simulink model "AFE_3L_DCP_DCN"  (R2013b)
settings: Solver=FixedStepDiscrete  SolverMode=SingleTasking  StartTime=0.0  StopTime=0.9  FixedStep=Tpas  RelTol=1e-3
values from neighbouring files (symbols this model uses):
  ASF3 = .5    (= 0.5)    [AFE_FV_Params.m]    (also in AFE_FV_ParamsPV4.m; Params.m)
  Cbus = 330e-3    (= 0.33)    [AFE_FV_Params.m]    (also in AFE_FV_ParamsPV4.m; Params.m)
  DAFE = 0    [AFE_FV_Params.m]    (also in AFE_FV_ParamsPV4.m; Params.m)
  fmod4Q = 1e3    (= 1000)    [AFE_FV_Params.m]    (also in AFE_FV_ParamsPV4.m; Params.m)
  Freq = 50    [AFE_FV_Params.m]    (also in AFE_FV_ParamsPV4.m; Params.m)
  IAFE3L = (PAFE3L+Numd(2)/Dend(1))/Ts    [AFE_FV_Params.m]    (also in AFE_FV_ParamsPV4.m = (PAFE3L+NumdAFE(2)/DendAFE(1))/Ts; CalcPIAndFilters.m; Params.m = (PAFE3L+NumdAFE(2)/DendAFE(1))/Ts)
  IDCP = (PDCP+Numd(2)/Dend(1))/Tpas    [AFE_FV_Params.m]    (also in AFE_FV_ParamsPV4.m = (PDCP+Numd(2)/Dend(1))/Ts; CalcPIAndFilters.m = (PDCP+Numd(2)/Dend(1))/Ts; Params.m = (PDCP+Numd(2)/Dend(1))/Ts)
  Kac = 1/(Vac*sqrt(2/3))    [AFE_FV_Params.m]    (also in AFE_FV_ParamsPV4.m; Params.m)
  KLPDCP = mat2str(KLPDCP)    [CalcPIAndFilters.m]
  L = .1    (= 0.1)    [AFE_FV_Params.m]    (also in AFE_FV_ParamsPV4.m; Params.m)
  Lac = 8.1487e-04    (= 0.00081487)    [AFE_FV_Params.m]    (also in AFE_FV_ParamsPV4.m; Params.m)
  Lcoup = 1e-6    (= 1e-06)    [AFE_FV_Params.m]    (also in AFE_FV_ParamsPV4.m = 1e-05; Params.m = 1e-05)
  NAFE = 100    [AFE_FV_Params.m]    (also in AFE_FV_ParamsPV4.m; Params.m)
  PAFE3L = Numd(1)/Dend(1)    [AFE_FV_Params.m]    (also in AFE_FV_ParamsPV4.m = NumdAFE(1)/DendAFE(1); CalcPIAndFilters.m; Params.m = NumdAFE(1)/DendAFE(1))
  PDCP = Numd(1)/Dend(1)    [AFE_FV_Params.m]    (also in AFE_FV_ParamsPV4.m; CalcPIAndFilters.m; Params.m)
  R = .28    (= 0.28)    [AFE_FV_Params.m]    (also in AFE_FV_ParamsPV4.m; Params.m)
  Sat3 = 800    [AFE_FV_Params.m]
  TLPDCP = mat2str(TLPDCP)    [CalcPIAndFilters.m]
  Tpas = 1e-6    (= 1e-06)    [AFE_FV_Params.m]    (also in AFE_FV_ParamsPV4.m; Params.m = 1e-05)
  Vac = 2000    [AFE_FV_Params.m]    (also in AFE_FV_ParamsPV4.m; Params.m)
  Vdc = 5000    [AFE_FV_Params.m]    (also in AFE_FV_ParamsPV4.m; Params.m)
undefined symbols (not defined in the file or in its folder): D1, Delta, Rac
libraries: powerlib x80, simulink x36, powerlib_meascontrol x26
(part 1 of 2)
settings Model: Creator=LiberT  LastModifiedBy=LiberT
settings DataIOCC: SignalLoggingSaveFormat=ModelDataLogs
settings OptimizationCC: ExpressionDepthLimit=2147483647
settings DebuggingCC: MultiTaskDSMMsg=warning  MultiTaskCondExecSysMsg=none  FcnCallInpInsideContextMsg=EnableAllAsWarning  StateNameClashWarn=warning
settings RTWCC: IncludeERTFirstTime=on

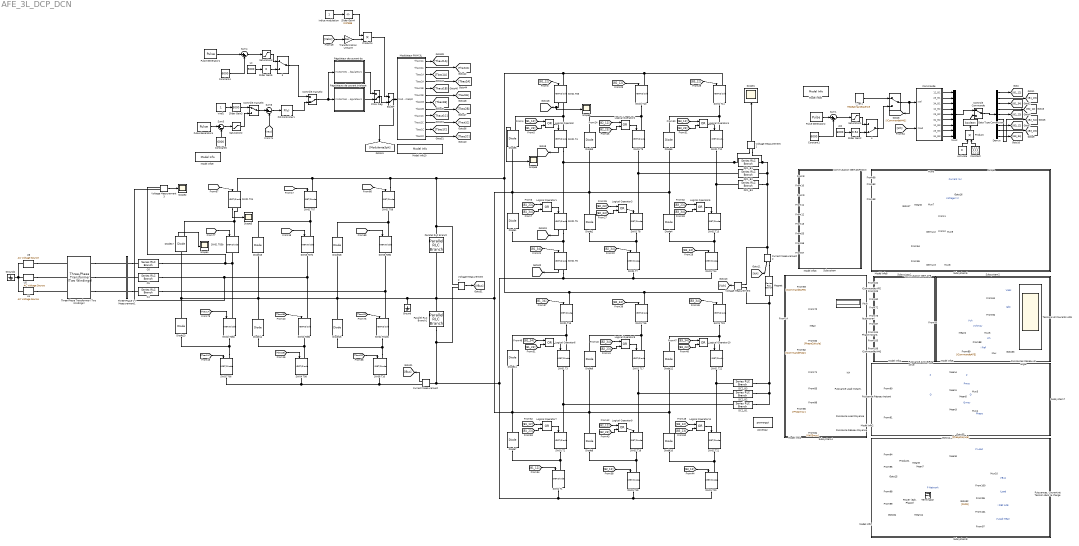
== system AFE_3L_DCP_DCN ==
  " " : ManualSwitch
  " 3" : ManualSwitch
  " 4" : ManualSwitch  CurrentSetting=0
  Activate : Constant  Value=0
  BO/BF : ManualSwitch  CurrentSetting=0
  C4 : powerlib/Elements/Series RLC Branch  LConnTagsString=__new0  RConnTagsString=__new0  BranchType=L  Resistance=Rac  Inductance=Lac  SetiL0=off  InitialCurrent=0  Capacitance=300e-3  Setx0=off  InitialVoltage=0  Measurements=None
  C5 : powerlib/Elements/Series RLC Branch  LConnTagsString=__new0  RConnTagsString=__new0  BranchType=L  Resistance=Rac  Inductance=Lac  SetiL0=off  InitialCurrent=0  Capacitance=300e-3  Setx0=off  InitialVoltage=0  Measurements=None
  C6 : powerlib/Elements/Series RLC Branch  LConnTagsString=__new0  RConnTagsString=__new0  BranchType=L  Resistance=Rac  Inductance=Lac  SetiL0=off  InitialCurrent=0  Capacitance=300e-3  Setx0=off  InitialVoltage=0  Measurements=None
  Choix Reg : ManualSwitch  CurrentSetting=0
  Commande : Subsystem
  Commutation IGBT AFE : Scope  NumInputPorts=9
      settings: TickLabels=on  TimeRange=0.04  YMin=-0.2~-0.2~-0.2~-0.2~-0.2~-0.2~-5~-5~-5  YMax=1.2~1.2~1.2~1.2~1.2~1.2~5~5~5  SaveName=ScopeData4
  Commutation IGBT DCP-DCN : Scope  NumInputPorts=9
      settings: TickLabels=on  TimeRange=0.04  YMin=-0.2~-0.2~-0.2~-0.2~-0.2~-0.2~-0.2~-0.2~-0.2  YMax=1.2~1.2~1.2~1.2~1.2~1.2~1.2~1.2~1.2
  Constant : Constant  Value=[1 1 1 1 1 1 1 1 1]
  Constant1 : Constant  Value=6000
  Constant4 : Constant  Value=6000
  Constant5 : Constant  Value=6000
  Controle Commande : ManualSwitch
  Contrôle manuel2 : ManualSwitch  CurrentSetting=0
  Contrôle manuel3 : ManualSwitch
  Current Measurement : powerlib/Measurements/Current Measurement  PhasorSimulation=off  OutputType=Complex  PSBequivalent=0
  Current Measurement2 : powerlib/Measurements/Current Measurement  PhasorSimulation=off  OutputType=Complex  PSBequivalent=0
  DC1_B1 : powerlib/Elements/Series RLC Branch  LConnTagsString=__new0  RConnTagsString=__new0  BranchType=L  Resistance=0  Inductance=Lcoup  SetiL0=off  InitialCurrent=0  Capacitance=1e-6  Setx0=off  InitialVoltage=0  Measurements=Branch current
  DC1_B2 : powerlib/Elements/Series RLC Branch  LConnTagsString=__new0  RConnTagsString=__new0  BranchType=L  Resistance=0  Inductance=Lcoup  SetiL0=off  InitialCurrent=0  Capacitance=1e-6  Setx0=off  InitialVoltage=0  Measurements=Branch current
  DC1_B3 : powerlib/Elements/Series RLC Branch  LConnTagsString=__new0  RConnTagsString=__new0  BranchType=L  Resistance=0  Inductance=Lcoup  SetiL0=off  InitialCurrent=0  Capacitance=1e-6  Setx0=off  InitialVoltage=0  Measurements=Branch current
  "DC2_B1 " : powerlib/Elements/Series RLC Branch  LConnTagsString=__new0  RConnTagsString=__new0  BranchType=L  Resistance=0  Inductance=Lcoup  SetiL0=off  InitialCurrent=0  Capacitance=1e-6  Setx0=off  InitialVoltage=0  Measurements=Branch current
  DC2_B2 : powerlib/Elements/Series RLC Branch  LConnTagsString=__new0  RConnTagsString=__new0  BranchType=L  Resistance=0  Inductance=Lcoup  SetiL0=off  InitialCurrent=0  Capacitance=1e-6  Setx0=off  InitialVoltage=0  Measurements=Branch current
  DC2_B3 : powerlib/Elements/Series RLC Branch  LConnTagsString=__new0  RConnTagsString=__new0  BranchType=L  Resistance=0  Inductance=Lcoup  SetiL0=off  InitialCurrent=0  Capacitance=1e-6  Setx0=off  InitialVoltage=0  Measurements=Branch current
  Data Type Conversion : DataTypeConversion  OutDataTypeStr=boolean
  Demux : Demux  Outputs=9
  Demux2 : Demux  Outputs=2
  Demux3 : Demux  Outputs=2
  Diode{1..4,6..16,18} (16 alike) : powerlib/Power Electronics/Diode  Ron=0.001  Lon=0  Vf=0.8  IC=0  UseSnubber=off  Rs=500  Cs=inf  Measurements=off
  Diode17 : powerlib/Power Electronics/Diode  Ron=0.001  Lon=0  Vf=0.8  IC=0  UseSnubber=off  Rs=500  Cs=inf  Measurements=on
  Diode5 : powerlib/Power Electronics/Diode  Ron=0.001  Lon=0  Vf=0.8  IC=0  UseSnubber=off  Rs=500  Cs=inf  Measurements=on
  Ground : powerlib/Elements/Ground  LConnTagsString=a
  Ground2 : powerlib/Elements/Ground  LConnTagsString=a
  "ICommande AFE " : Display
  ICommande H4Q : Display
  Ibusmoyen : Display
  Ich : Display
  Logical Operator{,1..11} (12 alike) : Logic  Operator=OR  AllPortsSameDT=off  OutDataTypeStr=boolean
  Magnet : powerlib/Elements/Series RLC Branch  LConnTagsString=__new0  RConnTagsString=__new0  BranchType=RL  Resistance=R  Inductance=L  SetiL0=off  InitialCurrent=0  Capacitance=1e-6  Setx0=off  InitialVoltage=0  Measurements=Branch voltage and current
  Mean{,1..3,8} (5 alike) : powerlib_meascontrol/Measurements/Mean  Freq=50  Vinit=0  Ts=Tpas
  Mean11 : powerlib_meascontrol/Measurements/Mean  Freq=1/.9  Vinit=0  Ts=Tpas
  Mean4 : powerlib_meascontrol/Measurements/Mean  Freq=fmod4Q*3  Vinit=0  Ts=Tpas
  Mean5 : powerlib_meascontrol/Measurements/Mean  Freq=fmod4Q*3  Vinit=0  Ts=Tpas
  Mean6 : powerlib_meascontrol/Measurements/Mean  Freq=fmod4Q/3  Vinit=0  Ts=Tpas
  Mean7 : powerlib_meascontrol/Measurements/Mean  Freq=1/.9  Vinit=0  Ts=Tpas
  Mean9 : powerlib_meascontrol/Measurements/Mean  Freq=fmod4Q/2  Vinit=0  Ts=Tpas
  Model Info{1..5,7..8} (7 alike) : simulink/Model-Wide Utilities/Model Info  InitialBlockCM=None  BlockCM=None  Frame=on  DisplayStringWithTags=Résultats  HorizontalTextAlignment=Center  LeftAlignmentValue=0.5  SourceBlockDiagram=AFE_3L_DCP_DCN  TagMaxNumber=20
  Model Info10 : simulink/Model-Wide Utilities/Model Info  InitialBlockCM=None  BlockCM=None  Frame=on  DisplayStringWithTags=Commande onduleur NPC3L  HorizontalTextAlignment=Center  LeftAlignmentValue=0.5  SourceBlockDiagram=AFE_3L_DCP_DCN  TagMaxNumber=20
  Model Info6 : simulink/Model-Wide Utilities/Model Info  InitialBlockCM=None  BlockCM=None  Frame=on  DisplayStringWithTags=Commande H4Q  HorizontalTextAlignment=Center  LeftAlignmentValue=0.5  SourceBlockDiagram=AFE_3L_DCP_DCN  TagMaxNumber=20
  Model Info9 : simulink/Model-Wide Utilities/Model Info  InitialBlockCM=None  BlockCM=None  Frame=on  DisplayStringWithTags=Commande AFE  HorizontalTextAlignment=Center  LeftAlignmentValue=0.5  SourceBlockDiagram=AFE_3L_DCP_DCN  TagMaxNumber=20
  Modulateur PWM 3L : Subsystem
  Mux{,3..10} (9 alike) : Mux  Inputs=2
  Mux2 : Mux  Inputs=9
  PID Controller1 : simulink/Continuous/PID Controller  Controller=PI  TimeDomain=Discrete-time  SampleTime=Tpas  IntegratorMethod=Forward Euler  FilterMethod=Forward Euler  Form=Parallel  P=PAFE3L  I=IAFE3L  D=0  N=100  InitialConditionSource=internal  InitialConditionForIntegrator=0  InitialConditionForFilter=0  ExternalReset=none  LimitOutput=on  UpperSaturationLimit=Sat3  LowerSaturationLimit=-Sat3  LinearizeAsGain=on  AntiWindupMode=clamping  Kb=1  TrackingMode=off  Kt=1  PParamMin=[]  PParamMax=[]  IParamMin=[]  IParamMax=[]  DParamMin=[]  DParamMax=[]  NParamMin=[]  NParamMax=[]  KbParamMin=[]  KbParamMax=[]  KtParamMin=[]  KtParamMax=[]  POutMin=[]  POutMax=[]  IOutMin=[]  IOutMax=[]  DOutMin=[]  DOutMax=[]  NOutMin=[]  NOutMax=[]  KbOutMin=[]  KbOutMax=[]  KtOutMin=[]  KtOutMax=[]  IntegratorOutMin=[]  IntegratorOutMax=[]  FilterOutMin=[]  FilterOutMax=[]  SumOutMin=[]  SumOutMax=[]  SumI1OutMin=[]  SumI1OutMax=[]  SumI2OutMin=[]  SumI2OutMax=[]  SumI3OutMin=[]  SumI3OutMax=[]  SumDOutMin=[]  SumDOutMax=[]  SaturationOutMin=[]  SaturationOutMax=[]  IntegratorContinuousStateAttributes=''  IntegratorStateMustResolveToSignalObject=off  IntegratorRTWStateStorageClass=Auto  FilterContinuousStateAttributes=''  FilterStateMustResolveToSignalObject=off  FilterRTWStateStorageClass=Auto
  Parallel RLC Branch : powerlib/Elements/Parallel RLC Branch  LConnTagsString=a  RConnTagsString=__new0  BranchType=C  Resistance=9.26  Inductance=1e-3  SetiL0=off  InitialCurrent=0  Capacitance=Cbus*2  Setx0=on  InitialVoltage=Vdc/2  Measurements=None
  Parallel RLC Branch1 : powerlib/Elements/Parallel RLC Branch  LConnTagsString=a  RConnTagsString=__new0  BranchType=C  Resistance=9.26  Inductance=1e-3  SetiL0=off  InitialCurrent=0  Capacitance=Cbus*2  Setx0=on  InitialVoltage=Vdc/2  Measurements=None
  Phase instant. : Display
  "Power (3ph, Phasor)" : powerlib_meascontrol/Measurements/Power (3ph, Phasor)
  Product : Product
  Product1 : Product
  Product4 : Product
  Puissance Active/Reactive : Subsystem
  Puissance Load Instant. : Display
  Puissance Load Moyenne : Display
  Puissance Réseau Instant : Display
  Puissance Réseau Moyenne : Display
  Puissances Réseau et angle : Scope  NumInputPorts=3
      settings: TickLabels=on  TimeRange=0.04  YMin=750000~-400000~-6  YMax=4e+06~250000~10  SaveName=ScopeData2
  "Puissances, Courant et Tension dans la charge" : Scope  NumInputPorts=5
      settings: TickLabels=on  ShowLegends=on  TimeRange=0.9  YMin=2e+06~4650~2000~755~1750  YMax=1.1e+07~5000~4000~800~3250  SaveName=ScopeData7
  Pulse Generator1 : DiscretePulseGenerator  Amplitude=12000  Period=floor(.4/Tpas)  PulseWidth=floor(.4/2/Tpas)  SampleTime=Tpas
  Pulse Generator2 : DiscretePulseGenerator  Amplitude=12000  Period=floor(.4 /Tpas)  PulseWidth=floor(.4 * .5 / Tpas)  PhaseDelay=floor(.001 / Tpas)  SampleTime=Tpas
  Pulse Generator4 : DiscretePulseGenerator  Amplitude=12000  Period=floor(.2/Tpas)  PulseWidth=floor(.2/2/Tpas)  SampleTime=Tpas
  Régulateur de courant dq : Subsystem
  Régulateurs de courant triphasé : Subsystem
  SW01 T05 : powerlib/Power Electronics/IGBT//Diode  Ron=Ron  Rs=Rs  Cs=Cs  Measurements=on
  SW01 T05b : powerlib/Power Electronics/IGBT//Diode  Ron=1e-3  Rs=1e5  Cs=Tpas  Measurements=off
  SW01 T07 : powerlib/Power Electronics/IGBT//Diode  Ron=1e-3  Rs=1e5  Cs=Tpas  Measurements=off
  SW01 T09 : powerlib/Power Electronics/IGBT//Diode  Ron=1e-3  Rs=1e5  Cs=Tpas  Measurements=off
  SW01 T{1..3,7..23} (20 alike) : powerlib/Power Electronics/IGBT//Diode  Ron=Ron  Rs=Rs  Cs=Cs  Measurements=off
  SW01 T24 : powerlib/Power Electronics/IGBT//Diode  Ron=1e-3  Rs=1e5  Cs=Tpas  Measurements=on
  SW01 T4 : powerlib/Power Electronics/IGBT//Diode  Ron=Ron  Rs=Rs  Cs=Cs  Measurements=on
  SW01 T5 : powerlib/Power Electronics/IGBT//Diode  Ron=Ron  Rs=Rs  Cs=Cs  Measurements=on
  SW01 T6 : powerlib/Power Electronics/IGBT//Diode  Ron=Ron  Rs=Rs  Cs=Cs  Measurements=on
  SW02 T010b : powerlib/Power Electronics/IGBT//Diode  Ron=1e-3  Rs=1e5  Cs=Tpas  Measurements=off
  SW02 T06 : powerlib/Power Electronics/IGBT//Diode  Ron=1e-3  Rs=1e5  Cs=Tpas  Measurements=off
  SW02 T06b : powerlib/Power Electronics/IGBT//Diode  Ron=1e-3  Rs=1e5  Cs=Tpas  Measurements=off
  SW02 T08b : powerlib/Power Electronics/IGBT//Diode  Ron=1e-3  Rs=1e5  Cs=Tpas  Measurements=off
  SW03 T07b : powerlib/Power Electronics/IGBT//Diode  Ron=1e-3  Rs=1e5  Cs=Tpas  Measurements=off
  SW04 T08 : powerlib/Power Electronics/IGBT//Diode  Ron=1e-3  Rs=1e5  Cs=Tpas  Measurements=off
  SW05 T09b : powerlib/Power Electronics/IGBT//Diode  Ron=1e-3  Rs=1e5  Cs=Tpas  Measurements=off
  SW06 T10 : powerlib/Power Electronics/IGBT//Diode  Ron=1e-3  Rs=1e5  Cs=Tpas  Measurements=off
  Saturation1 : Saturate  UpperLimit=5000  LowerLimit=2000
  Saturation2 : Saturate  UpperLimit=5500  LowerLimit=4800
  Saturation3 : Saturate  UpperLimit=5000  LowerLimit=1000
  Scope : Scope  NumInputPorts=6
      settings: TimeRange=0.9  YMin=-7000~-5000~-0.1~-0.1~-15000~0  YMax=7000~5000~1.1~1.1~15000~2500  SaveName=hash  MaxDataPoints=10000
  Scope{1..6} (6 alike) : Scope
      Scope1 settings: TimeRange=0.9  YMin=-7000  YMax=7000  SaveName=ScopeData6  MaxDataPoints=10000
      Scope2 settings: YMin=-5500  YMax=5500  SaveName=PHPH
      Scope3 settings: YMin=-1250  YMax=2750  SaveName=IGBTA
      Scope4 settings: YMin=-5500  YMax=5500  SaveName=DIODEA
      Scope5 settings: YMin=-5500  YMax=5500  SaveName=IGBTH
      Scope6 settings: YMin=-5500  YMax=5500  SaveName=DIODEH
  Slider Gain2 : simulink/Math Operations/Slider Gain  low=0  gain=0.54  high=1
  Slider Gain3 : simulink/Math Operations/Slider Gain  low=0  gain=5000  high=7000
  Slider Gain4 : simulink/Math Operations/Slider Gain  low=0  gain=0.97696  high=1
  Slider Gain5 : simulink/Math Operations/Slider Gain  low=0  gain=0  high=1
  Subsystem : Subsystem
      mask Display: disp('')
  Subsystem1 : Subsystem
      mask Display: disp('')
  Subsystem2 : Subsystem
      mask Display: disp('')
  Subsystem4 : Subsystem
      mask Display: disp('')
  Subsystem6 : Subsystem
      mask Display: disp('')
  Subsystem7 : Subsystem
      mask Display: disp('')
  Subsystem8 : Subsystem
      mask Display: disp('')
  Sum{1,4..6} (4 alike) : Sum  Inputs=|+-
  Tensions et Courants AFE : Scope  NumInputPorts=4
      settings: TickLabels=on  ShowLegends=on  TimeRange=0.04  YMin=-2000~-750~4999.4~-800  YMax=2000~750~5000.1~600  SaveName=hach4quadrants
  Terminator : Terminator
  Three-Phase Transformer (Two Windings) : powerlib/Elements/Three-Phase Transformer (Two Windings)  Winding1Connection=Delta (D1)  UNITS=pu  NominalPower=[ 2500e3 , 50 ]  Winding1=[ 18000 , 0 , 0 ]  Winding2Connection=Yg  Winding2=[ 2000 , 0 , 0 ]  SetSaturation=off  Rm=500  Lm=500  Saturation=[ 0,0 ; 0.0024,1.2 ; 1.0,1.52 ]  Hysteresis=off  DataFile='hysteresis'  SetInitialFlux=off  InitialFluxes=[ 0.8 , -0.8 , 0.7 ]  Measurements=None  MoreParameters=off  BreakLoop=off  DataType=off  TransfoNumber=1
  Three-Phase V-I Measurement1 : powerlib/Measurements/Three-Phase V-I Measurement  VoltageMeasurement=phase-to-ground  SetLabelV=on  LabelV=Vabc  Vpu=off  VpuLL=off  CurrentMeasurement=yes  SetLabelI=on  LabelI=Iabc  Ipu=off  Pbase=100e6  Vbase=500e3  OutputType=Complex  PhasorSimulation=off  PSBequivalent=0
  Transformation Unitaire : Gain  Gain=Kac
  U4 : powerlib/Electrical Sources/AC Voltage Source  Amplitude=Vac*sqrt(2/3)*9  Phase=120  Frequency=Freq  SampleTime=Tpas  Measurements=Voltage
  U5 : powerlib/Electrical Sources/AC Voltage Source  Amplitude=Vac*sqrt(2/3)*9  Phase=-120  Frequency=Freq  SampleTime=Tpas  Measurements=Voltage
  U6 : powerlib/Electrical Sources/AC Voltage Source  Amplitude=Vac*sqrt(2/3)*9  Phase=0  Frequency=Freq  SampleTime=Tpas  Measurements=Voltage
  Vbus : Display
  Voltage Measurement{,1..3} (4 alike) : powerlib/Measurements/Voltage Measurement  PhasorSimulation=off  OutputType=Complex  PSBequivalent=0
  Vref1 : Constant  SampleTime=Tpas
  i_ref 1 : simulink/Sources/Repeating Sequence  rep_seq_t="[0 108.51e-3 127.6e-3 132e-3 200e-3 250e-3 283.33e-3 310e-3 366.66e-3  490e-3 533e-3 683.33e-3 900e-3]"  rep_seq_y=[333 333 1000 1031 1500 2000 2500 3000 4000 6000 6000 333 333]
  indice modulation : Constant
  powergui : powerlib/powergui  Priority=1  SimulationMode=Discrete  SolverType=Tustin  SampleTime=Tpas  frequency=60  SPID=off  DisableSnubberDevices=off  DisableRonSwitches=off  DisableVfSwitches=off  SwTol=0  Interpol=off  DisplayEquations=off  frequencyindice=50  Pbase=100e6  ErrMax=1e-4  Iterations=50  UnitsV=kV  UnitsW=MW  FunctionMessages=off  echomessages=off  HookPort=off  EnableUseOfTLC=off  x0status=blocks  RestoreLinks=warning  ResistiveCurrentMeasurement=off  Frange=[0:2:500]  Ylog=off  Xlog=on  ShowGrid=off  save=off  variable=ZData  structure=ScopeData1  ZoomFFT=off  StartTime=18  cycles=100  DisplayStyle=1  fundamental=50  FreqAxis=off  MaxFrequency=2000  frequencyindicesteady=1  RmsSteady=1  display=off  Ts=0  methode=off
  uo : Constant  Value=5000
  uo2 : Constant  Value=6000
  wires:
  [B1_12] -> Commutation IGBT DCP-DCN/1
  [B1_23] -> Commutation IGBT DCP-DCN/2
  [B1_34] -> Commutation IGBT DCP-DCN/3
  [B2_12] -> Commutation IGBT DCP-DCN/4
  [B2_23] -> Commutation IGBT DCP-DCN/5
  [B2_34] -> Commutation IGBT DCP-DCN/6
  Constant/1 -> Product/2
  Activate/1 -> Product/1
  Controle Commande/1 -> Demux/1
  Mux2/1 -> Controle Commande/1
  Data Type Conversion/1 -> Controle Commande/2
  Product/1 -> Data Type Conversion/1
  Demux/1 -> [B1_12]
  Demux/3 -> [B1_34]
  Demux/2 -> [B1_23]
  [B1_12] -> SW01 T05/1
  Logical Operator/1 -> SW01 T4/1
  [B1_12] -> Logical Operator/1
  [B1_23] -> Logical Operator/2
  Logical Operator1/1 -> SW01 T5/1
  [B1_23] -> Logical Operator1/1
  [B1_34] -> Logical Operator1/2
  [B1_34] -> SW01 T6/1
  [B2_12] -> SW01 T10/1
  Logical Operator2/1 -> SW01 T9/1
  [B2_12] -> Logical Operator2/1
  [B2_23] -> Logical Operator2/2
  Logical Operator3/1 -> SW01 T8/1
  [B2_23] -> Logical Operator3/1
  [B2_34] -> Logical Operator3/2
  [B2_34] -> SW01 T7/1
  [B3_12] -> SW01 T11/1
  Logical Operator4/1 -> SW01 T12/1
  [B3_12] -> Logical Operator4/1
  [B3_23] -> Logical Operator4/2
  Logical Operator5/1 -> SW01 T13/1
  [B3_23] -> Logical Operator5/1
  [B3_34] -> Logical Operator5/2
  [B3_34] -> SW01 T14/1
  [B1_34] -> SW01 T15/1
  Logical Operator6/1 -> SW01 T3/1
  [B1_34] -> Logical Operator6/1
  [B1_23] -> Logical Operator6/2
  Logical Operator7/1 -> SW01 T2/1
  [B1_12] -> Logical Operator7/1
  [B1_23] -> Logical Operator7/2
  [B1_12] -> SW01 T1/1
  [B2_34] -> SW01 T16/1
  Logical Operator8/1 -> SW01 T17/1
  [B2_34] -> Logical Operator8/1
  [B2_23] -> Logical Operator8/2
  Logical Operator9/1 -> SW01 T18/1
  [B2_12] -> Logical Operator9/1
  [B2_23] -> Logical Operator9/2
  [B2_12] -> SW01 T19/1
  [B3_34] -> SW01 T23/1
  Logical Operator10/1 -> SW01 T22/1
  [B3_34] -> Logical Operator10/1
  [B3_23] -> Logical Operator10/2
  Logical Operator11/1 -> SW01 T21/1
  [B3_12] -> Logical Operator11/1
  [B3_23] -> Logical Operator11/2
  [B3_12] -> SW01 T20/1
  uo2/1 -> Slider Gain2/1
  Slider Gain2/1 -> " 4"/2
  Saturation1/1 -> " 4"/1
  Constant1/1 -> Sum1/2
  i_ref 1/1 -> " "/1
  " 4"/1 -> " "/2
  Pulse Generator2/1 -> Sum1/1
  Sum1/1 -> Saturation1/1
  " "/1 -> Commande/1(Iref), [ICommandeH4Q]
  Demux/4 -> [B2_12]
  Demux/6 -> [B2_34]
  Demux/5 -> [B2_23]
  Demux/7 -> [B3_12]
  Demux/9 -> [B3_34]
  Demux/8 -> [B3_23]
  Current Measurement2/1 -> [Ich]
  Voltage Measurement/1 -> [Vch]
  [B3_12] -> Commutation IGBT DCP-DCN/7
  [B3_23] -> Commutation IGBT DCP-DCN/8
  [B3_34] -> Commutation IGBT DCP-DCN/9
  Mux6/1 -> [ILoadScope], Scope/1  "Current (A)"
  Mux7/1 -> Scope/2  "Voltage (V)"
  [Ich] -> Mux6/2
  [mIGBT1] -> Demux2/1
  Mean6/1 -> [VMeanLoad], Mux7/2
  [Vch] -> Mux7/1, Mean6/1
  [mIGBT2] -> Demux3/1
  [B1_12] -> Scope/3
  Mux8/1 -> Scope/6
  Mux9/1 -> Scope/5
  [B1_34] -> Scope/4
  Demux2/1 -> Mux9/1
  Demux3/1 -> Mux9/2
  Demux2/2 -> Mux8/1
  Demux3/2 -> Mux8/2
  [ICommandeH4Q] -> Mux6/1
  SW01 T4/1 -> [mIGBT2]
  SW01 T05/1 -> Scope5/1, [mIGBT1]
  SW01 T5/1 -> [mIGBT3]
  SW01 T6/1 -> [mIGBT4]
  Voltage Measurement1/1 -> Scope1/1
  Current Measurement/1 -> [IBus]
  [Thaut1A] -> SW01 T24/1
  [Tbas1A] -> SW02 T06b/1
  [Tbas2A] -> SW02 T06/1
  [Thaut1B] -> SW01 T07/1
  [Thaut2B] -> SW03 T07b/1
  [Tbas1B] -> SW02 T08b/1
  [Tbas2B] -> SW04 T08/1
  [Thaut1C] -> SW01 T09/1
  [Thaut2C] -> SW05 T09b/1
  [Tbas1C] -> SW02 T010b/1
  [Tbas2C] -> SW06 T10/1
  Voltage Measurement2/1 -> [VBus]
  Mean/1 -> Ibusmoyen/1
  [VBus] -> Vbus/1
  [IBus] -> Mean/1
  [ICommandeAFE] -> "ICommande AFE "/1
  [PhaseCalcule] -> Phase instant./1
  [PAFEmoy] -> Puissance Réseau Moyenne/1
  [PH4Q] -> Puissance Load Instant./1
  [Ich] -> Ich/1
  [ICommandeH4Q] -> ICommande H4Q/1
  [PAFE] -> Puissance Réseau Instant/1
  [PH4Qmoy] -> Puissance Load Moyenne/1
  [T5] -> Commutation IGBT AFE/1
  [T56] -> Commutation IGBT AFE/2
  [T6] -> Commutation IGBT AFE/3
  [T7] -> Commutation IGBT AFE/4
  [T78] -> Commutation IGBT AFE/5
  [T8] -> Commutation IGBT AFE/6
  [Vabc] -> Tensions et Courants AFE/1  "Vabc"
  [Iabc] -> Tensions et Courants AFE/2  "Iabc"
  [IBus] -> Mux/1  "Ich"
  [ICommandeAFE] -> Mux/2  "I Ref"
  Mux/1 -> [IBusScope], Tensions et Courants AFE/4
  [Vabc] -> Puissance Active/Reactive/1(Vabc)
  [Iabc] -> Puissance Active/Reactive/2(Iabc)
  Puissance Active/Reactive/1(P) -> Mean4/1, Mean1/1  "P"
  Puissance Active/Reactive/2(Q) -> Mean3/1, Mean5/1  "Q"
  Puissance Active/Reactive/3(PhC) -> Puissances Réseau et angle/3, [PhaseCalcule]  "Phase"
  Mean1/1 -> Mux3/2  "Pmoy"
  Mux3/1 -> Puissances Réseau et angle/1
  Mean3/1 -> Mux4/2  "Qmoy"
  Mux4/1 -> Puissances Réseau et angle/2
  Mux5/1 -> Tensions et Courants AFE/3
  [VBus] -> Mux5/1, Mean2/1  "Vch"
  Mean2/1 -> Mux5/2  "Vchmoy"
  Mean4/1 -> Mux3/1  "P"
  Mean5/1 -> Mux4/1  "Q"
  Mean7/1 -> [PH4Qmoy]
  [Vch] -> Product1/1
  [Ich] -> Product1/2
  Product1/1 -> Mean9/1
  Mean9/1 -> Mean7/1, Mean8/1
  Mean8/1 -> [PH4Q], Mux10/1  "P Load"
  [VMeanLoad] -> "Puissances, Courant et Tension dans la charge"/5  "VLoad Mean"
  Mux10/1 -> "Puissances, Courant et Tension dans la charge"/1
  [VBus] -> "Puissances, Courant et Tension dans la charge"/2  "VBus"
  [ILoadScope] -> "Puissances, Courant et Tension dans la charge"/3  "ILoad"
  [ICommandeAFE] -> "Puissances, Courant et Tension dans la charge"/4  "I REF AFE"
  [Vabc] -> "Power (3ph, Phasor)"/1
  [Iabc] -> "Power (3ph, Phasor)"/2
  Mean11/1 -> [PAFEmoy]
  [T9] -> Commutation IGBT AFE/7
  [T910] -> Commutation IGBT AFE/8
  [T100] -> Commutation IGBT AFE/9
  Commande/1(12_B1) -> Mux2/1
  Commande/2(23_B1) -> Mux2/2
  Commande/3(34_B1) -> Mux2/3
  Commande/4(12_B2) -> Mux2/4
  Commande/5(23_B2) -> Mux2/5
  Commande/6(34_B2) -> Mux2/6
  Commande/7(12_B3) -> Mux2/7
  Commande/8(23_B3) -> Mux2/8
  [Ich] -> Commande/2("Iload ")
  Commande/9(34_B3) -> Mux2/9
  Voltage Measurement3/1 -> Scope2/1
  [Thaut2A] -> SW01 T05b/1
  [VBus] -> Sum6/2
  Vref1/1 -> Slider Gain3/1
  Sum6/1 -> PID Controller1/1
  PID Controller1/1 -> Contrôle manuel2/2
  Contrôle manuel2/1 -> Régulateur de courant dq/1(In1), Régulateurs de courant triphasé/1(In1)
  Sum5/1 -> Saturation2/1
  Pulse Generator4/1 -> Sum5/1
  Constant5/1 -> Sum5/2
  Contrôle manuel3/1 -> Sum6/1
  Slider Gain3/1 -> Contrôle manuel3/1
  Saturation2/1 -> Contrôle manuel3/2
  Modulateur PWM 3L/1(Thaut1A) -> [Thaut1A]
  Modulateur PWM 3L/2(Thaut2A) -> [Thaut2A]
  Modulateur PWM 3L/3(Tbas1A) -> [Tbas1A]
  Modulateur PWM 3L/4(Tbas2A) -> [Tbas2A]
  Modulateur PWM 3L/5(Thaut1B) -> [Thaut1B]
  Modulateur PWM 3L/6(Thaut2B) -> [Thaut2B]
  Modulateur PWM 3L/7(Tbas1B) -> [Tbas1B]
  Modulateur PWM 3L/8(Tbas2B) -> [Tbas2B]
  Modulateur PWM 3L/9(Thaut1C) -> [Thaut1C]
  Modulateur PWM 3L/10(Thaut2C) -> [Thaut2C]
  Modulateur PWM 3L/11(Tbas1C) -> [Tbas1C]
  Modulateur PWM 3L/12(Tbas2C) -> [Tbas2C]
  indice modulation/1 -> Slider Gain4/1
  [Vabc] -> Transformation Unitaire/1
  Transformation Unitaire/1 -> Product4/2
  Slider Gain4/1 -> Product4/1
  BO/BF/1 -> [Modulante3ph], Modulateur PWM 3L/1(Modulante3ph)
  uo/1 -> Slider Gain5/1
  " 3"/1 -> Contrôle manuel2/1
  Slider Gain5/1 -> " 3"/2
  Saturation3/1 -> " 3"/1
  Sum4/1 -> Saturation3/1
  Pulse Generator1/1 -> Sum4/1
  Constant4/1 -> Sum4/2
  Choix Reg/1 -> BO/BF/2
  Régulateurs de courant triphasé/1(Sorties Régulateurs) -> Choix Reg/2
  Régulateur de courant dq/1(Sorties Régulateurs) -> Choix Reg/1
  Product4/1 -> BO/BF/1
  "Power (3ph, Phasor)"/2 -> Terminator/1
  "Power (3ph, Phasor)"/1 -> [PAFE], Mux10/2  "P Network"
  SW01 T24/1 -> Scope3/1
  Diode17/1 -> Scope4/1
  Diode5/1 -> Scope6/1
  connections:
  DC1_B1/LConn1 -- SW01 T5/LConn1 -- SW01 T4/RConn1 -- Voltage Measurement1/LConn1
  DC1_B3/LConn1 -- SW01 T13/LConn1 -- SW01 T12/RConn1
  DC1_B2/LConn1 -- SW01 T9/RConn1 -- SW01 T8/LConn1
  Diode5/RConn1 -- SW01 T05/RConn1 -- SW01 T4/LConn1
  Diode3/RConn1 -- SW01 T10/RConn1 -- SW01 T9/LConn1
  Diode6/RConn1 -- SW01 T12/LConn1 -- SW01 T11/RConn1
  Diode1/LConn1 -- SW01 T6/LConn1 -- SW01 T5/RConn1
  Diode4/LConn1 -- SW01 T14/LConn1 -- SW01 T13/RConn1
  Diode2/LConn1 -- SW01 T8/RConn1 -- SW01 T7/LConn1
  Parallel RLC Branch1/RConn1 -- Voltage Measurement2/LConn2 -- Current Measurement/LConn1 -- SW01 T1/RConn1 -- SW01 T20/RConn1 -- SW01 T19/RConn1 -- SW01 T6/RConn1 -- SW01 T14/RConn1 -- SW01 T7/RConn1
  SW01 T09/LConn1 -- Voltage Measurement2/LConn1 -- Parallel RLC Branch/LConn1 -- SW01 T11/LConn1 -- SW01 T10/LConn1 -- SW01 T05/LConn1 -- SW01 T23/LConn1 -- SW01 T16/LConn1 -- SW01 T15/LConn1 -- SW01 T24/LConn1 -- SW01 T07/LConn1
  Diode11/RConn1 -- SW01 T15/RConn1 -- SW01 T3/LConn1
  Diode9/RConn1 -- SW01 T17/LConn1 -- SW01 T16/RConn1
  Diode12/RConn1 -- SW01 T23/RConn1 -- SW01 T22/LConn1
  Diode7/LConn1 -- SW01 T2/RConn1 -- SW01 T1/LConn1
  Diode10/LConn1 -- SW01 T21/RConn1 -- SW01 T20/LConn1
  Diode8/LConn1 -- SW01 T19/LConn1 -- SW01 T18/RConn1
  Diode13/RConn1 -- Diode17/LConn1 -- Diode15/LConn1 -- Diode14/RConn1 -- Diode16/RConn1 -- Diode18/LConn1 -- Ground/LConn1 -- Parallel RLC Branch1/LConn1 -- Diode11/LConn1 -- Diode7/RConn1 -- Diode9/LConn1 -- Diode8/RConn1 -- Diode10/RConn1 -- Diode12/LConn1 -- Diode4/RConn1 -- Diode6/LConn1 -- Diode3/LConn1 -- Diode2/RConn1 -- Diode5/LConn1 -- Diode1/RConn1 -- Parallel RLC Branch/RConn1
  SW01 T21/LConn1 -- DC2_B3/RConn1 -- SW01 T22/RConn1
  SW01 T2/LConn1 -- "DC2_B1 "/RConn1 -- SW01 T3/RConn1
  SW01 T17/RConn1 -- DC2_B2/RConn1 -- SW01 T18/LConn1
  DC1_B1/RConn1 -- Voltage Measurement/LConn1 -- Current Measurement2/LConn1 -- DC1_B3/RConn1 -- DC1_B2/RConn1 -- Voltage Measurement1/LConn2
  DC2_B3/LConn1 -- "DC2_B1 "/LConn1 -- DC2_B2/LConn1 -- Voltage Measurement/LConn2 -- Magnet/RConn1
  Current Measurement2/RConn1 -- Magnet/LConn1
  C6/LConn1 -- Voltage Measurement3/LConn1 -- SW02 T06b/LConn1 -- SW01 T05b/RConn1
  SW05 T09b/RConn1 -- SW02 T010b/LConn1 -- C4/LConn1
  SW03 T07b/RConn1 -- Voltage Measurement3/LConn2 -- C5/LConn1 -- SW02 T08b/LConn1
  SW01 T24/RConn1 -- SW01 T05b/LConn1 -- Diode17/RConn1
  SW01 T07/RConn1 -- SW03 T07b/LConn1 -- Diode15/RConn1
  SW01 T09/RConn1 -- SW05 T09b/LConn1 -- Diode18/RConn1
  SW02 T06/LConn1 -- SW02 T06b/RConn1 -- Diode13/LConn1
  SW06 T10/LConn1 -- SW02 T010b/RConn1 -- Diode16/LConn1
  SW02 T08b/RConn1 -- SW04 T08/LConn1 -- Diode14/LConn1
  SW04 T08/RConn1 -- SW02 T06/RConn1 -- SW06 T10/RConn1 -- Current Measurement/RConn1
  U5/LConn1 -- Ground2/LConn1 -- U4/LConn1 -- U6/LConn1
  C5/RConn1 -- Three-Phase V-I Measurement1/LConn2
  Three-Phase V-I Measurement1/LConn3 -- C4/RConn1
  U6/RConn1 -- Three-Phase Transformer (Two Windings)/LConn1
  Three-Phase Transformer (Two Windings)/RConn1 -- Three-Phase V-I Measurement1/RConn1
  U5/RConn1 -- Three-Phase Transformer (Two Windings)/LConn2
  Three-Phase Transformer (Two Windings)/RConn2 -- Three-Phase V-I Measurement1/RConn2
  U4/RConn1 -- Three-Phase Transformer (Two Windings)/LConn3
  Three-Phase Transformer (Two Windings)/RConn3 -- Three-Phase V-I Measurement1/RConn3
  Three-Phase V-I Measurement1/LConn1 -- C6/RConn1

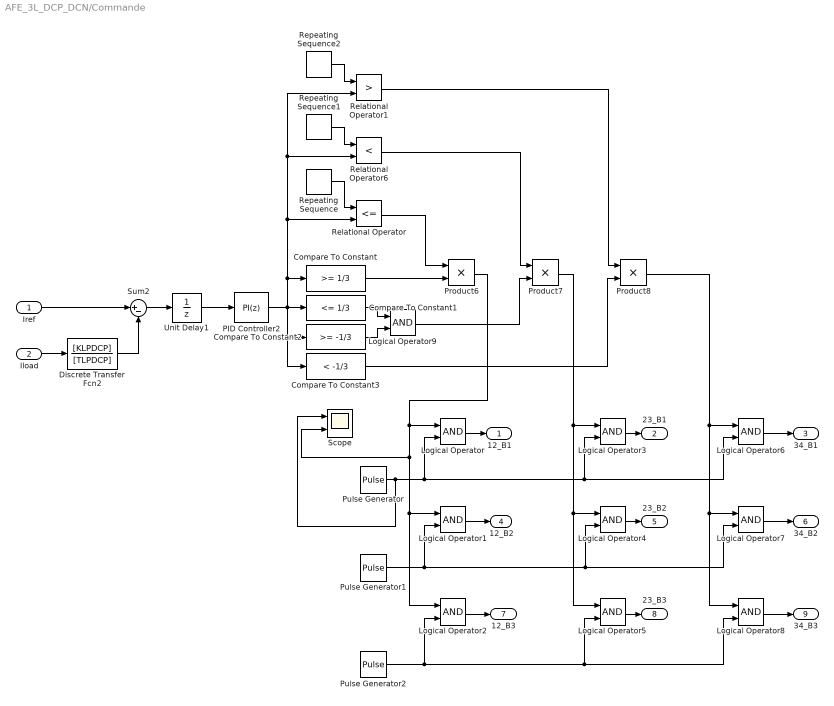
== system AFE_3L_DCP_DCN/Commande ==
  Iref : Inport
  "Iload " : Inport  Port=2
  Compare To Constant : simulink/Logic and Bit Operations/Compare To Constant  relop=>=  const=1/3  OutDataTypeStr=boolean
  Compare To Constant1 : simulink/Logic and Bit Operations/Compare To Constant  relop=<=  const=1/3  OutDataTypeStr=boolean
  Compare To Constant2 : simulink/Logic and Bit Operations/Compare To Constant  relop=>=  const=-1/3  OutDataTypeStr=boolean
  Compare To Constant3 : simulink/Logic and Bit Operations/Compare To Constant  relop=<  const=-1/3  OutDataTypeStr=boolean
  Discrete Transfer Fcn2 : DiscreteTransferFcn  Numerator=[KLPDCP]  Denominator=[TLPDCP]  SampleTime=Tpas
  Logical Operator{,1..9} (10 alike) : Logic  AllPortsSameDT=off  OutDataTypeStr=boolean  SampleTime=Tpas
  PID Controller2 : simulink/Continuous/PID Controller  Controller=PI  TimeDomain=Discrete-time  SampleTime=Tpas  IntegratorMethod=Forward Euler  FilterMethod=Forward Euler  Form=Parallel  P=PDCP  I=IDCP  D=0  N=100  InitialConditionSource=internal  InitialConditionForIntegrator=0  InitialConditionForFilter=0  ExternalReset=none  LimitOutput=on  UpperSaturationLimit=1  LowerSaturationLimit=-1  LinearizeAsGain=on  AntiWindupMode=clamping  Kb=1  TrackingMode=off  Kt=1  PParamMin=[]  PParamMax=[]  IParamMin=[]  IParamMax=[]  DParamMin=[]  DParamMax=[]  NParamMin=[]  NParamMax=[]  KbParamMin=[]  KbParamMax=[]  KtParamMin=[]  KtParamMax=[]  POutMin=[]  POutMax=[]  IOutMin=[]  IOutMax=[]  DOutMin=[]  DOutMax=[]  NOutMin=[]  NOutMax=[]  KbOutMin=[]  KbOutMax=[]  KtOutMin=[]  KtOutMax=[]  IntegratorOutMin=[]  IntegratorOutMax=[]  FilterOutMin=[]  FilterOutMax=[]  SumOutMin=[]  SumOutMax=[]  SumI1OutMin=[]  SumI1OutMax=[]  SumI2OutMin=[]  SumI2OutMax=[]  SumI3OutMin=[]  SumI3OutMax=[]  SumDOutMin=[]  SumDOutMax=[]  SaturationOutMin=[]  SaturationOutMax=[]  IntegratorContinuousStateAttributes=''  IntegratorStateMustResolveToSignalObject=off  IntegratorRTWStateStorageClass=Auto  FilterContinuousStateAttributes=''  FilterStateMustResolveToSignalObject=off  FilterRTWStateStorageClass=Auto
  Product6 : Product  SampleTime=Tpas
  Product7 : Product  SampleTime=Tpas
  Product8 : Product  SampleTime=Tpas
  Pulse Generator : DiscretePulseGenerator  Period=floor(1/(fmod4Q/3) * 1/Tpas)  PulseWidth=floor(1/(fmod4Q) * 1/Tpas)  SampleTime=Tpas
  Pulse Generator1 : DiscretePulseGenerator  Period=floor(1/(fmod4Q/3) * 1/Tpas)  PulseWidth=floor(1/(fmod4Q) * 1/Tpas)  PhaseDelay=floor(1/(fmod4Q) * 1/Tpas)  SampleTime=Tpas
  Pulse Generator2 : DiscretePulseGenerator  Period=floor(1/(fmod4Q/3) * 1/Tpas)  PulseWidth=floor(1/(fmod4Q) * 1/Tpas)  PhaseDelay=floor(2/(fmod4Q) * 1/Tpas)  SampleTime=Tpas
  Relational Operator : RelationalOperator  Operator=<=  OutDataTypeStr=boolean
  Relational Operator1 : RelationalOperator  Operator=>  OutDataTypeStr=boolean
  Relational Operator6 : RelationalOperator  Operator=<  OutDataTypeStr=boolean
  Repeating Sequence : simulink/Sources/Repeating Sequence  rep_seq_t=[0 1/fmod4Q]  rep_seq_y=[1/3 1.035]
  Repeating Sequence1 : simulink/Sources/Repeating Sequence  rep_seq_t=[0 1/fmod4Q]  rep_seq_y=[-.35 .35]
  Repeating Sequence2 : simulink/Sources/Repeating Sequence  rep_seq_t=[0 1/fmod4Q]  rep_seq_y=[-1 -1/3]
  Scope : Scope  NumInputPorts=2
      settings: YMin=-5~-5  YMax=5~5  SaveName=aaaaa
  Sum2 : Sum  Inputs=|+-
  Unit Delay1 : UnitDelay  SampleTime=-1
  12_B1 : Outport
  23_B1 : Outport  Port=2
  34_B1 : Outport  Port=3
  12_B2 : Outport  Port=4
  23_B2 : Outport  Port=5
  34_B2 : Outport  Port=6
  12_B3 : Outport  Port=7
  23_B3 : Outport  Port=8
  34_B3 : Outport  Port=9
  wires:
  Compare To Constant/1 -> Product6/2
  Compare To Constant3/1 -> Product8/2
  Compare To Constant1/1 -> Logical Operator9/1
  Compare To Constant2/1 -> Logical Operator9/2
  Logical Operator9/1 -> Product7/2
  Repeating Sequence/1 -> Relational Operator/1
  Repeating Sequence2/1 -> Relational Operator1/1
  Relational Operator/1 -> Product6/1
  Relational Operator6/1 -> Product7/1
  Relational Operator1/1 -> Product8/1
  PID Controller2/1 -> Relational Operator/2, Relational Operator1/2, Relational Operator6/2, Compare To Constant/1, Compare To Constant1/1, Compare To Constant3/1, Compare To Constant2/1
  Repeating Sequence1/1 -> Relational Operator6/1
  Iref/1 -> Sum2/1
  "Iload "/1 -> Discrete Transfer Fcn2/1
  Discrete Transfer Fcn2/1 -> Sum2/2
  Sum2/1 -> Unit Delay1/1
  Unit Delay1/1 -> PID Controller2/1
  Product6/1 -> Scope/2, Logical Operator2/1, Logical Operator1/1, Logical Operator/1
  Pulse Generator2/1 -> Logical Operator5/2, Logical Operator8/2, Logical Operator2/2
  Pulse Generator/1 -> Scope/1, Logical Operator3/2, Logical Operator6/2, Logical Operator/2
  Pulse Generator1/1 -> Logical Operator1/2, Logical Operator4/2, Logical Operator7/2
  Product7/1 -> Logical Operator5/1, Logical Operator4/1, Logical Operator3/1
  Product8/1 -> Logical Operator8/1, Logical Operator7/1, Logical Operator6/1
  Logical Operator/1 -> 12_B1/1
  Logical Operator8/1 -> 34_B3/1
  Logical Operator1/1 -> 12_B2/1
  Logical Operator3/1 -> 23_B1/1
  Logical Operator6/1 -> 34_B1/1
  Logical Operator2/1 -> 12_B3/1
  Logical Operator5/1 -> 23_B3/1
  Logical Operator7/1 -> 34_B2/1
  Logical Operator4/1 -> 23_B2/1

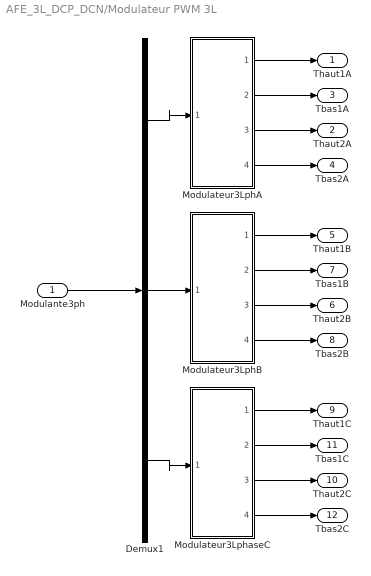
== system AFE_3L_DCP_DCN/Modulateur PWM 3L ==
  Modulante3ph : Inport
  Demux1 : Demux  Outputs=3
  "Modulateur3LphA " : Subsystem
  Modulateur3LphB : Subsystem
  Modulateur3LphaseC : Subsystem
  Thaut1A : Outport
  Thaut2A : Outport  Port=2
  Tbas1A : Outport  Port=3
  Tbas2A : Outport  Port=4
  Thaut1B : Outport  Port=5
  Thaut2B : Outport  Port=6
  Tbas1B : Outport  Port=7
  Tbas2B : Outport  Port=8
  Thaut1C : Outport  Port=9
  Thaut2C : Outport  Port=10
  Tbas1C : Outport  Port=11
  Tbas2C : Outport  Port=12
  wires:
  Modulante3ph/1 -> Demux1/1
  Demux1/1 -> "Modulateur3LphA "/1(Modulante)
  "Modulateur3LphA "/1(Thaut1) -> Thaut1A/1
  "Modulateur3LphA "/2(Tbas1) -> Tbas1A/1
  "Modulateur3LphA "/3(Thaut2) -> Thaut2A/1
  "Modulateur3LphA "/4(Tbas2) -> Tbas2A/1
  Demux1/2 -> Modulateur3LphB/1(Modulante)
  Modulateur3LphB/1(Thaut1) -> Thaut1B/1
  Modulateur3LphB/2(Tbas1) -> Tbas1B/1
  Modulateur3LphB/3(Thaut2) -> Thaut2B/1
  Modulateur3LphB/4(Tbas2) -> Tbas2B/1
  Demux1/3 -> Modulateur3LphaseC/1(Modulante)
  Modulateur3LphaseC/1(Thaut1) -> Thaut1C/1
  Modulateur3LphaseC/2(Tbas1) -> Tbas1C/1
  Modulateur3LphaseC/3(Thaut2) -> Thaut2C/1
  Modulateur3LphaseC/4(Tbas2) -> Tbas2C/1

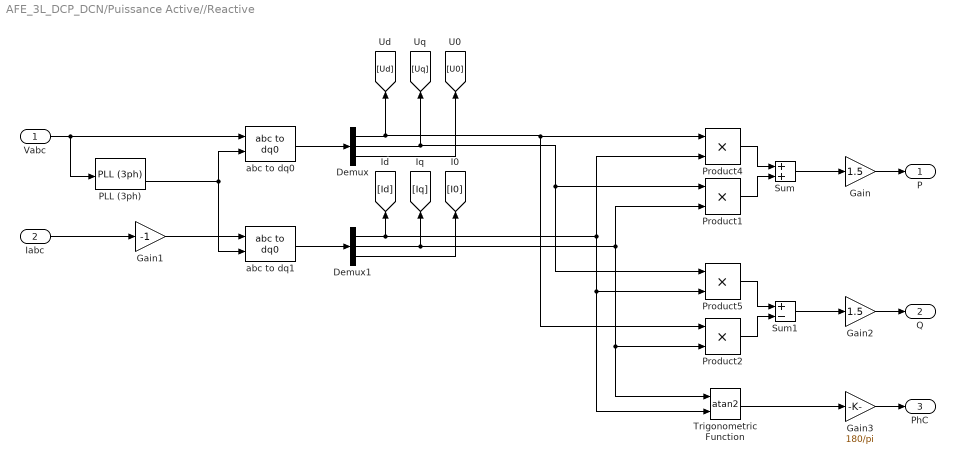
== system AFE_3L_DCP_DCN/Puissance Active//Reactive ==
  Vabc : Inport
  Iabc : Inport  Port=2
  Demux : Demux  Outputs=3
  Demux1 : Demux  Outputs=3
  Gain : Gain  Gain=1.5
  Gain1 : Gain  Gain=-1
  Gain2 : Gain  Gain=1.5
  Gain3 : Gain  Gain=180/pi
  PLL (3ph) : powerlib_meascontrol/PLL/PLL (3ph)  Fmin=49  Par_Init=[0, 50]  ParK=[180, 3200, 1]  TcD=1e-4  MaxRateChangeFreq=6  FilterCutOffFreq=25  Ts=Tpas  AGC=on
  Product{1..2,4..5} (4 alike) : Product
  Sum : Sum
  Sum1 : Sum  Inputs=+-
  Trigonometric Function : Trigonometry  Operator=atan2
  abc to dq0 : powerlib_meascontrol/Transformations/abc to dq0  Alignment=90 degrees behind phase A axis
  abc to dq1 : powerlib_meascontrol/Transformations/abc to dq0  Alignment=90 degrees behind phase A axis
  P : Outport
  Q : Outport  Port=2
  PhC : Outport  Port=3
  wires:
  Vabc/1 -> PLL (3ph)/1, abc to dq0/1
  abc to dq0/1 -> Demux/1
  abc to dq1/1 -> Demux1/1
  Product2/1 -> Sum1/2
  Sum1/1 -> Gain2/1
  Demux/3 -> [U0]
  Demux/2 -> Product5/1, Product1/1, [Uq]
  Demux/1 -> Product2/1, Product4/1, [Ud]
  Demux1/2 -> [Iq], Trigonometric Function/1, Product2/2, Product1/2
  Product5/1 -> Sum1/1
  Gain2/1 -> Q/1
  Trigonometric Function/1 -> Gain3/1
  Gain3/1 -> PhC/1
  Product4/1 -> Sum/1
  Product1/1 -> Sum/2
  Sum/1 -> Gain/1
  Gain/1 -> P/1
  Demux1/1 -> [Id], Trigonometric Function/2, Product5/2, Product4/2
  Demux1/3 -> [I0]
  PLL (3ph)/2 -> abc to dq1/2, abc to dq0/2
  Iabc/1 -> Gain1/1
  Gain1/1 -> abc to dq1/1

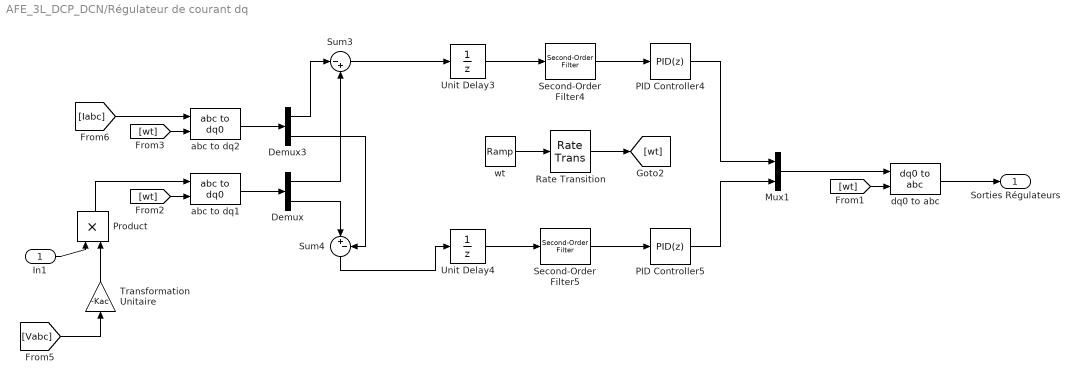
== system AFE_3L_DCP_DCN/Régulateur de courant dq ==
  In1 : Inport
  Demux : Demux  Outputs=2
  Demux3 : Demux  Outputs=2
  Mux1 : Mux  Inputs=2
  PID Controller4 : simulink/Continuous/PID Controller  Controller=PID  TimeDomain=Discrete-time  SampleTime=Tpas  IntegratorMethod=Forward Euler  FilterMethod=Forward Euler  Form=Parallel  P=PAFE3L  I=IAFE3L  D=DAFE  N=NAFE  InitialConditionSource=internal  InitialConditionForIntegrator=0  InitialConditionForFilter=0  ExternalReset=none  LimitOutput=on  UpperSaturationLimit=0.95  LowerSaturationLimit=-0.95  LinearizeAsGain=on  AntiWindupMode=clamping  Kb=1  TrackingMode=off  Kt=1  PParamMin=[]  PParamMax=[]  IParamMin=[]  IParamMax=[]  DParamMin=[]  DParamMax=[]  NParamMin=[]  NParamMax=[]  KbParamMin=[]  KbParamMax=[]  KtParamMin=[]  KtParamMax=[]  POutMin=[]  POutMax=[]  IOutMin=[]  IOutMax=[]  DOutMin=[]  DOutMax=[]  NOutMin=[]  NOutMax=[]  KbOutMin=[]  KbOutMax=[]  KtOutMin=[]  KtOutMax=[]  IntegratorOutMin=[]  IntegratorOutMax=[]  FilterOutMin=[]  FilterOutMax=[]  SumOutMin=[]  SumOutMax=[]  SumI1OutMin=[]  SumI1OutMax=[]  SumI2OutMin=[]  SumI2OutMax=[]  SumI3OutMin=[]  SumI3OutMax=[]  SumDOutMin=[]  SumDOutMax=[]  SaturationOutMin=[]  SaturationOutMax=[]  IntegratorContinuousStateAttributes=''  IntegratorStateMustResolveToSignalObject=off  IntegratorRTWStateStorageClass=Auto  FilterContinuousStateAttributes=''  FilterStateMustResolveToSignalObject=off  FilterRTWStateStorageClass=Auto
  PID Controller5 : simulink/Continuous/PID Controller  Controller=PID  TimeDomain=Discrete-time  SampleTime=Tpas  IntegratorMethod=Forward Euler  FilterMethod=Forward Euler  Form=Parallel  P=PAFE3L  I=IAFE3L  D=DAFE  N=NAFE  InitialConditionSource=internal  InitialConditionForIntegrator=0  InitialConditionForFilter=0  ExternalReset=none  LimitOutput=on  UpperSaturationLimit=0.95  LowerSaturationLimit=-0.95  LinearizeAsGain=on  AntiWindupMode=clamping  Kb=1  TrackingMode=off  Kt=1  PParamMin=[]  PParamMax=[]  IParamMin=[]  IParamMax=[]  DParamMin=[]  DParamMax=[]  NParamMin=[]  NParamMax=[]  KbParamMin=[]  KbParamMax=[]  KtParamMin=[]  KtParamMax=[]  POutMin=[]  POutMax=[]  IOutMin=[]  IOutMax=[]  DOutMin=[]  DOutMax=[]  NOutMin=[]  NOutMax=[]  KbOutMin=[]  KbOutMax=[]  KtOutMin=[]  KtOutMax=[]  IntegratorOutMin=[]  IntegratorOutMax=[]  FilterOutMin=[]  FilterOutMax=[]  SumOutMin=[]  SumOutMax=[]  SumI1OutMin=[]  SumI1OutMax=[]  SumI2OutMin=[]  SumI2OutMax=[]  SumI3OutMin=[]  SumI3OutMax=[]  SumDOutMin=[]  SumDOutMax=[]  SaturationOutMin=[]  SaturationOutMax=[]  IntegratorContinuousStateAttributes=''  IntegratorStateMustResolveToSignalObject=off  IntegratorRTWStateStorageClass=Auto  FilterContinuousStateAttributes=''  FilterStateMustResolveToSignalObject=off  FilterRTWStateStorageClass=Auto
  Product : Product
  Rate Transition : RateTransition  OutPortSampleTime=Ts
  Second-Order Filter4 : powerlib_meascontrol/Filters/Second-Order Filter  FilterType=Lowpass  Fo=ASF3*fmod4Q  Zeta=QSF3  Ts=Tpas  Initialize=on  Vac_Init="[0,  0,  50]"  Vdc_Init=0  PlotResponse=off  FreqRange=[0, 10000, 1]
  Second-Order Filter5 : powerlib_meascontrol/Filters/Second-Order Filter  FilterType=Lowpass  Fo=ASF3*fmod4Q  Zeta=QSF3  Ts=Tpas  Initialize=on  Vac_Init="[0,  0,  50]"  Vdc_Init=0  PlotResponse=off  FreqRange=[0, 10000, 1]
  Sum3 : Sum  Inputs=|-+
  Sum4 : Sum  Inputs=|+-
  Transformation Unitaire : Gain  Gain=-Kac
  Unit Delay3 : UnitDelay  SampleTime=-1
  Unit Delay4 : UnitDelay  SampleTime=-1
  abc to dq1 : powerlib_meascontrol/Transformations/abc to dq0  Alignment=Aligned with phase A axis
  abc to dq2 : powerlib_meascontrol/Transformations/abc to dq0  Alignment=Aligned with phase A axis
  dq0 to abc : powerlib_meascontrol/Transformations/dq0 to abc  Alignment=Aligned with phase A axis
  wt : simulink/Sources/Ramp  slope=2*pi*50  start=0  X0=0
  Sorties Régulateurs : Outport
  wires:
  [Vabc] -> Transformation Unitaire/1
  Transformation Unitaire/1 -> Product/2
  In1/1 -> Product/1
  abc to dq1/1 -> Demux/1
  [wt] -> abc to dq1/2
  [wt] -> dq0 to abc/2
  wt/1 -> Rate Transition/1
  Rate Transition/1 -> [wt]
  Mux1/1 -> dq0 to abc/1
  Sum3/1 -> Unit Delay3/1
  PID Controller4/1 -> Mux1/1
  Demux/1 -> Sum3/2
  [Iabc] -> abc to dq2/1
  [wt] -> abc to dq2/2
  abc to dq2/1 -> Demux3/1
  Demux3/1 -> Sum3/1
  Product/1 -> abc to dq1/1
  Sum4/1 -> Unit Delay4/1
  PID Controller5/1 -> Mux1/2
  dq0 to abc/1 -> Sorties Régulateurs/1
  Unit Delay3/1 -> Second-Order Filter4/1
  Second-Order Filter4/1 -> PID Controller4/1
  Unit Delay4/1 -> Second-Order Filter5/1
  Second-Order Filter5/1 -> PID Controller5/1
  Demux/2 -> Sum4/1
  Demux3/2 -> Sum4/2

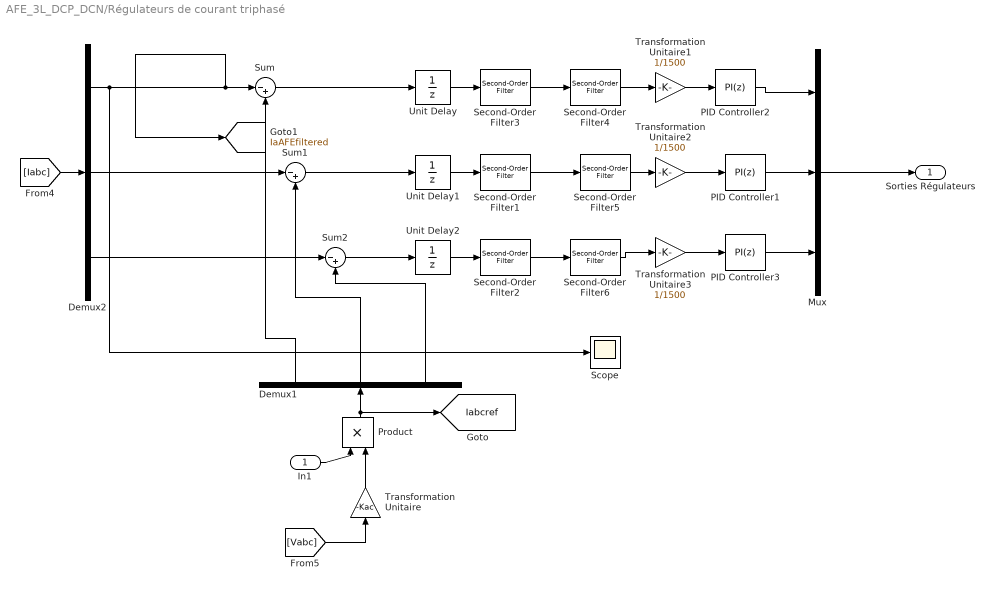
== system AFE_3L_DCP_DCN/Régulateurs de courant triphasé ==
  In1 : Inport
  Demux1 : Demux  Outputs=3
  Demux2 : Demux  Outputs=3
  Mux : Mux  Inputs=3
  PID Controller1 : simulink/Continuous/PID Controller  Controller=PI  TimeDomain=Discrete-time  SampleTime=Tpas  IntegratorMethod=Forward Euler  FilterMethod=Forward Euler  Form=Parallel  P=PDCP  I=IDCP  D=DAFE  N=NAFE  InitialConditionSource=internal  InitialConditionForIntegrator=0  InitialConditionForFilter=0  ExternalReset=none  LimitOutput=on  UpperSaturationLimit=0.95  LowerSaturationLimit=-0.95  LinearizeAsGain=on  AntiWindupMode=clamping  Kb=1  TrackingMode=off  Kt=1  PParamMin=[]  PParamMax=[]  IParamMin=[]  IParamMax=[]  DParamMin=[]  DParamMax=[]  NParamMin=[]  NParamMax=[]  KbParamMin=[]  KbParamMax=[]  KtParamMin=[]  KtParamMax=[]  POutMin=[]  POutMax=[]  IOutMin=[]  IOutMax=[]  DOutMin=[]  DOutMax=[]  NOutMin=[]  NOutMax=[]  KbOutMin=[]  KbOutMax=[]  KtOutMin=[]  KtOutMax=[]  IntegratorOutMin=[]  IntegratorOutMax=[]  FilterOutMin=[]  FilterOutMax=[]  SumOutMin=[]  SumOutMax=[]  SumI1OutMin=[]  SumI1OutMax=[]  SumI2OutMin=[]  SumI2OutMax=[]  SumI3OutMin=[]  SumI3OutMax=[]  SumDOutMin=[]  SumDOutMax=[]  SaturationOutMin=[]  SaturationOutMax=[]  IntegratorContinuousStateAttributes=''  IntegratorStateMustResolveToSignalObject=off  IntegratorRTWStateStorageClass=Auto  FilterContinuousStateAttributes=''  FilterStateMustResolveToSignalObject=off  FilterRTWStateStorageClass=Auto
  PID Controller2 : simulink/Continuous/PID Controller  Controller=PI  TimeDomain=Discrete-time  SampleTime=Tpas  IntegratorMethod=Forward Euler  FilterMethod=Forward Euler  Form=Parallel  P=PDCP  I=IDCP  D=DAFE  N=NAFE  InitialConditionSource=internal  InitialConditionForIntegrator=0  InitialConditionForFilter=0  ExternalReset=none  LimitOutput=on  UpperSaturationLimit=0.95  LowerSaturationLimit=-0.95  LinearizeAsGain=on  AntiWindupMode=clamping  Kb=1  TrackingMode=off  Kt=1  PParamMin=[]  PParamMax=[]  IParamMin=[]  IParamMax=[]  DParamMin=[]  DParamMax=[]  NParamMin=[]  NParamMax=[]  KbParamMin=[]  KbParamMax=[]  KtParamMin=[]  KtParamMax=[]  POutMin=[]  POutMax=[]  IOutMin=[]  IOutMax=[]  DOutMin=[]  DOutMax=[]  NOutMin=[]  NOutMax=[]  KbOutMin=[]  KbOutMax=[]  KtOutMin=[]  KtOutMax=[]  IntegratorOutMin=[]  IntegratorOutMax=[]  FilterOutMin=[]  FilterOutMax=[]  SumOutMin=[]  SumOutMax=[]  SumI1OutMin=[]  SumI1OutMax=[]  SumI2OutMin=[]  SumI2OutMax=[]  SumI3OutMin=[]  SumI3OutMax=[]  SumDOutMin=[]  SumDOutMax=[]  SaturationOutMin=[]  SaturationOutMax=[]  IntegratorContinuousStateAttributes=''  IntegratorStateMustResolveToSignalObject=off  IntegratorRTWStateStorageClass=Auto  FilterContinuousStateAttributes=''  FilterStateMustResolveToSignalObject=off  FilterRTWStateStorageClass=Auto
  PID Controller3 : simulink/Continuous/PID Controller  Controller=PI  TimeDomain=Discrete-time  SampleTime=Tpas  IntegratorMethod=Forward Euler  FilterMethod=Forward Euler  Form=Parallel  P=PDCP  I=IDCP  D=DAFE  N=NAFE  InitialConditionSource=internal  InitialConditionForIntegrator=0  InitialConditionForFilter=0  ExternalReset=none  LimitOutput=on  UpperSaturationLimit=0.95  LowerSaturationLimit=-0.95  LinearizeAsGain=on  AntiWindupMode=clamping  Kb=1  TrackingMode=off  Kt=1  PParamMin=[]  PParamMax=[]  IParamMin=[]  IParamMax=[]  DParamMin=[]  DParamMax=[]  NParamMin=[]  NParamMax=[]  KbParamMin=[]  KbParamMax=[]  KtParamMin=[]  KtParamMax=[]  POutMin=[]  POutMax=[]  IOutMin=[]  IOutMax=[]  DOutMin=[]  DOutMax=[]  NOutMin=[]  NOutMax=[]  KbOutMin=[]  KbOutMax=[]  KtOutMin=[]  KtOutMax=[]  IntegratorOutMin=[]  IntegratorOutMax=[]  FilterOutMin=[]  FilterOutMax=[]  SumOutMin=[]  SumOutMax=[]  SumI1OutMin=[]  SumI1OutMax=[]  SumI2OutMin=[]  SumI2OutMax=[]  SumI3OutMin=[]  SumI3OutMax=[]  SumDOutMin=[]  SumDOutMax=[]  SaturationOutMin=[]  SaturationOutMax=[]  IntegratorContinuousStateAttributes=''  IntegratorStateMustResolveToSignalObject=off  IntegratorRTWStateStorageClass=Auto  FilterContinuousStateAttributes=''  FilterStateMustResolveToSignalObject=off  FilterRTWStateStorageClass=Auto
  Product : Product
  Scope : Scope
      settings: TimeRange=0.04  YMin=-6000  YMax=6000  SaveName=ScopeData2
  Second-Order Filter{1..6} (6 alike) : powerlib_meascontrol/Filters/Second-Order Filter  FilterType=Lowpass  Fo=1.25*fmod4Q  Zeta=1  Ts=Tpas  Initialize=on  Vac_Init="[0,  0,  50]"  Vdc_Init=0  PlotResponse=off  FreqRange=[0, 10000, 1]
  Sum : Sum  Inputs=|-+
  Sum1 : Sum  Inputs=|-+
  Sum2 : Sum  Inputs=|-+
  Transformation Unitaire : Gain  Gain=-Kac
  Transformation Unitaire1 : Gain  Gain=1/1500
  Transformation Unitaire2 : Gain  Gain=1/1500
  Transformation Unitaire3 : Gain  Gain=1/1500
  Unit Delay : UnitDelay  SampleTime=-1
  Unit Delay1 : UnitDelay  SampleTime=-1
  Unit Delay2 : UnitDelay  SampleTime=-1
  Sorties Régulateurs : Outport
  tag scope: IaAFEfiltered=global, Iabcref=global
  wires:
  Sum/1 -> Unit Delay/1
  Sum1/1 -> Unit Delay1/1
  Sum2/1 -> Unit Delay2/1
  [Iabc] -> Demux2/1
  [Vabc] -> Transformation Unitaire/1
  Demux1/1 -> Sum/2
  Demux1/2 -> Sum1/2
  Demux1/3 -> Sum2/2
  Transformation Unitaire/1 -> Product/2
  In1/1 -> Product/1
  Product/1 -> Demux1/1, [Iabcref]
  PID Controller3/1 -> Mux/3
  PID Controller1/1 -> Mux/2
  PID Controller2/1 -> Mux/1
  Demux2/1 -> [IaAFEfiltered], Sum/1, Scope/1
  Demux2/2 -> Sum1/1
  Demux2/3 -> Sum2/1
  Second-Order Filter3/1 -> Second-Order Filter4/1
  Unit Delay/1 -> Second-Order Filter3/1
  Unit Delay1/1 -> Second-Order Filter1/1
  Second-Order Filter1/1 -> Second-Order Filter5/1
  Second-Order Filter2/1 -> Second-Order Filter6/1
  Unit Delay2/1 -> Second-Order Filter2/1
  Mux/1 -> Sorties Régulateurs/1
  Second-Order Filter4/1 -> Transformation Unitaire1/1
  Second-Order Filter5/1 -> Transformation Unitaire2/1
  Second-Order Filter6/1 -> Transformation Unitaire3/1
  Transformation Unitaire1/1 -> PID Controller2/1
  Transformation Unitaire2/1 -> PID Controller1/1
  Transformation Unitaire3/1 -> PID Controller3/1

== system AFE_3L_DCP_DCN/Subsystem ==

== system AFE_3L_DCP_DCN/Subsystem1 ==

== system AFE_3L_DCP_DCN/Subsystem2 ==

== system AFE_3L_DCP_DCN/Subsystem4 ==

== system AFE_3L_DCP_DCN/Subsystem6 ==

== system AFE_3L_DCP_DCN/Subsystem7 ==

== system AFE_3L_DCP_DCN/Subsystem8 ==

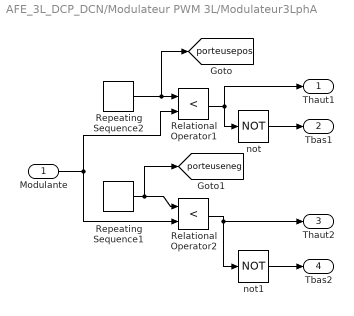
== system AFE_3L_DCP_DCN/Modulateur PWM 3L/Modulateur3LphA  ==
  Modulante : Inport
  Relational Operator1 : RelationalOperator  Operator=<  OutDataTypeStr=boolean
  Relational Operator2 : RelationalOperator  Operator=<  OutDataTypeStr=boolean
  Repeating Sequence1 : simulink/Sources/Repeating Sequence  rep_seq_t=[0 .5/(666) 1/(666)]  rep_seq_y=[-1 0 -1]
  Repeating Sequence2 : simulink/Sources/Repeating Sequence  rep_seq_t=[0 .5/(666) 1/(666)]  rep_seq_y=[0 1 0]
  not : Logic  Operator=NOT  IconShape=distinctive  AllPortsSameDT=off  OutDataTypeStr=boolean
  not1 : Logic  Operator=NOT  IconShape=distinctive  AllPortsSameDT=off  OutDataTypeStr=boolean
  Thaut1 : Outport
  Tbas1 : Outport  Port=2
  Thaut2 : Outport  Port=3
  Tbas2 : Outport  Port=4
  tag scope: porteuseneg=global, porteusepos=global
  wires:
  Repeating Sequence2/1 -> [porteusepos], Relational Operator1/1
  Modulante/1 -> Relational Operator1/2, Relational Operator2/2
  Repeating Sequence1/1 -> [porteuseneg], Relational Operator2/1
  Relational Operator1/1 -> not/1, Thaut1/1
  not/1 -> Tbas1/1
  not1/1 -> Tbas2/1
  Relational Operator2/1 -> not1/1, Thaut2/1
